simulink model "flightControlSystem"  (R2024b)
settings: Solver=ode3  StartTime=0  StopTime=TFinal  FixedStep=Ts  RelTol=1e-3  EnableMultiTasking=on
undefined symbols (not defined in the file): codertarget, Controller, DiscIntNeverNeededParam, Discrete, Estimator, g, gray, init, orient_ref, pos_ref, Sensors, Time, Ts, var_acc_angle_N, var_bias_gyr_N, var_gyro_p_N, Vehicle
libraries: simulink x42, slpidlib x6, simulink_extras x5, ctrlSharedLib x4, sharedtransform x3, visiontransforms x2, parrotlib x1, vrlib x1, visionanalysis x1, visionstatistics x1, visionconversions x1
(part 3 of 3)

== system flightControlSystem/Control System/State Estimator/SensorPreprocessing/sensordata_group ==
  HAL_acc_SI : Inport  OutDataTypeStr=Bus: HAL_acc_SI_t
  HAL_gyro_SI : Inport  Port=2  OutDataTypeStr=Bus: HAL_gyro_SI_t
  HAL_ultrasound_SI : Inport  Port=3  OutDataTypeStr=Bus: HAL_ultrasound_SI_t
  HAL_pressure_SI : Inport  Port=4  OutDataTypeStr=Bus: HAL_pressure_SI_t
  HAL_vbat_SI : Inport  Port=5  OutDataTypeStr=Bus: HAL_vbat_SI_t
  Bus Selector1 : BusSelector  OutputSignals=vbat_V,vbat_percentage
  Bus Selector3 : BusSelector  OutputSignals=x,y,z
  Bus Selector4 : BusSelector  OutputSignals=x,y,z,temperature
  Bus Selector5 : BusSelector  OutputSignals=altitude
  Bus Selector6 : BusSelector  OutputSignals=pressure
  Out Bus Element : Outport  VectorParamsAs1DForOutWhenUnconnected=off  PortName=sensordata_datin  Element=ddx
  Out Bus Element1 : Outport  VectorParamsAs1DForOutWhenUnconnected=off  PortName=sensordata_datin  Element=ddy
  Out Bus Element2 : Outport  VectorParamsAs1DForOutWhenUnconnected=off  PortName=sensordata_datin  Element=ddz
  Out Bus Element3 : Outport  VectorParamsAs1DForOutWhenUnconnected=off  PortName=sensordata_datin  Element=p
  Out Bus Element4 : Outport  VectorParamsAs1DForOutWhenUnconnected=off  PortName=sensordata_datin  Element=q
  Out Bus Element5 : Outport  VectorParamsAs1DForOutWhenUnconnected=off  PortName=sensordata_datin  Element=r
  Out Bus Element6 : Outport  VectorParamsAs1DForOutWhenUnconnected=off  PortName=sensordata_datin  Element=altitude_sonar
  Out Bus Element7 : Outport  VectorParamsAs1DForOutWhenUnconnected=off  PortName=sensordata_datin  Element=prs
  Out Bus Element8 : Outport  VectorParamsAs1DForOutWhenUnconnected=off  PortName=sensordata_datin  Element=vbat_V
  Out Bus Element9 : Outport  VectorParamsAs1DForOutWhenUnconnected=off  PortName=sensordata_datin  Element=vbat_percentage
  Out1 : Outport  Port=2
  wires:
  HAL_gyro_SI/1 -> Bus Selector4/1
  HAL_acc_SI/1 -> Bus Selector3/1
  HAL_pressure_SI/1 -> Bus Selector6/1
  HAL_ultrasound_SI/1 -> Bus Selector5/1
  Bus Selector4/1 -> Out Bus Element3/1  "<x>"
  Bus Selector3/3 -> Out Bus Element2/1  "<z>"
  Bus Selector4/3 -> Out Bus Element5/1  "<z>"
  Bus Selector5/1 -> Out Bus Element6/1  "<altitude>"
  Bus Selector6/1 -> Out Bus Element7/1  "<pressure>"
  Bus Selector4/2 -> Out Bus Element4/1  "<y>"
  Bus Selector3/1 -> Out Bus Element/1  "<x>"
  Bus Selector3/2 -> Out Bus Element1/1  "<y>"
  Bus Selector1/1 -> Out Bus Element8/1  "<vbat_V>"
  HAL_vbat_SI/1 -> Bus Selector1/1
  Bus Selector1/2 -> Out Bus Element9/1  "<vbat_percentage>"
  Bus Selector4/4 -> Out1/1  "<temperature>"

== system flightControlSystem/Control System/State Estimator/XY Position Estimator/EstimatorVelocity ==
  opticalFlow_datin : Inport
  Z_estimin : Inport  Port=2  SampleTime=Ts
  sensorIMU_datin : Inport  Port=3
  orient_estimin : Inport  Port=4
  angular velocity : Inport  Port=5
  AccelerationHandling : Subsystem
  Angular velocity compensation for optical flow : Subsystem
  DataHandling : Subsystem
  Delay : Delay  DelayLength=1  InitialCondition=0
  KalmanFilter_dxdy : ctrlSharedLib/Kalman Filter  TimeDomain=Discrete-Time  UseCurrentEstimator=on  ModelSource=Individual A, B, C, D matrices  ModelSourceVariable=ss(0.95,1,1,0,1)  A=Estimator.pos.kfVelo.A  B=Estimator.pos.kfVelo.B  C=Estimator.pos.kfVelo.C  D=Estimator.pos.kfVelo.D  NumberOfStates=1  NumberOfInputs=1  NumberOfOutputs=1  InitialEstimateSource=Dialog  X0=0  P0=10  UseK=off  UseGH=off  NumberOfProcessNoiseInputs=1  G=Estimator.pos.kfVelo.G  TimeInvariantG=on  H=Estimator.pos.kfVelo.H  TimeInvariantH=on  Q=Estimator.pos.kfVelo.Q  TimeInvariantQ=on  R=Estimator.pos.kfVelo.R  TimeInvariantR=on  N=Estimator.pos.kfVelo.N  TimeInvariantN=on  AddInputPort=on  AddEnablePort=on  OutputEstimatedY=off  OutputP=off  Ts=-1
  Selector1 : Selector  InputPortWidth=4  IndexOptions=Index vector (dialog)  Indices=[1 2]  OutputSizes=1
  Z_estimin1 : InportShadow  Port=2  SampleTime=Ts
  angular velocity compensation : Sum
  xy velocity w/o angular velocity compensation : Subsystem
  dxy_estimout : Outport  VectorParamsAs1DForOutWhenUnconnected=off
  wires:
  Z_estimin/1 -> DataHandling/1(Z_estimin), AccelerationHandling/4(Z_estimin)
  KalmanFilter_dxdy/1 -> Selector1/1
  sensorIMU_datin/1 -> AccelerationHandling/2(sensorIMU_datin), DataHandling/3(sensorIMU_datin)
  orient_estimin/1 -> AccelerationHandling/3(orient_estimin), DataHandling/2(orient_estimin)
  Z_estimin1/1 -> xy velocity w/o angular velocity compensation/2(z_estimate), Angular velocity compensation for optical flow/1(z_estimate)
  AccelerationHandling/1(acceleration_world) -> KalmanFilter_dxdy/1
  angular velocity compensation/1 -> KalmanFilter_dxdy/2
  Delay/1 -> DataHandling/5(dxyOF_datin)
  Selector1/1 -> dxy_estimout/1, Delay/1
  angular velocity/1 -> Angular velocity compensation for optical flow/2(Angular velocity w/o bias)
  Angular velocity compensation for optical flow/1(angular velocity correction) -> angular velocity compensation/2
  xy velocity w/o angular velocity compensation/1(optical_flow_dx_dy) -> DataHandling/4(dxy_estimin), AccelerationHandling/1(dxy_estimin), angular velocity compensation/1
  opticalFlow_datin/1 -> xy velocity w/o angular velocity compensation/1(optical_flow)
  DataHandling/1(enable_flag) -> KalmanFilter_dxdy/3

== system flightControlSystem/Control System/State Estimator/XY Position Estimator/EstimatorXYPosition ==
  note: Switching from orientationControl to Position
      | control reset the current world position estimate
      | (happens when using no markers)
  dxy_estimin : Inport
  orient_estimin : Inport  Port=2  SampleTime=Ts
  controlModePosVSOrient_flagin : Inport  Port=3
  dz_estimin : Inport  Port=4
  Math Function : Math  Operator=transpose  SignedPower=on
  Mux2 : Mux  Inputs=2
  Product : Product  Multiplication=Matrix(*)
  Rotation Angles to Direction Cosine Matrix : sharedtransform/Rotation Angles to Direction Cosine Matrix  rotationOrder=ZYX  aMode=aMode
  SelectdXY : Selector  InputPortWidth=3  IndexOptions=Index vector (dialog)  Indices=[1 2]  OutputSizes=1
  SimplyIntegrateVelocity : DiscreteIntegrator  ExternalReset=rising  SampleTime=Ts  ICPrevOutput=DiscIntNeverNeededParam  ICPrevScaledInput=DiscIntNeverNeededParam
  XY_estimout : Outport  VectorParamsAs1DForOutWhenUnconnected=off
  wires:
  controlModePosVSOrient_flagin/1 -> SimplyIntegrateVelocity/2
  Product/1 -> SelectdXY/1
  Mux2/1 -> Product/2
  dz_estimin/1 -> Mux2/2
  SimplyIntegrateVelocity/1 -> XY_estimout/1
  dxy_estimin/1 -> Mux2/1
  orient_estimin/1 -> Rotation Angles to Direction Cosine Matrix/1
  Rotation Angles to Direction Cosine Matrix/1 -> Math Function/1
  SelectdXY/1 -> SimplyIntegrateVelocity/1
  Math Function/1 -> Product/1

== system flightControlSystem/Control System/State Estimator/SensorPreprocessing/Temperature Compensation/Triggered Subsystem ==
  In1 : Inport
  Trigger : TriggerPort  TriggerType=either  VariantControl=Variant
  Out1 : Outport
  wires:
  In1/1 -> Out1/1

== system flightControlSystem/Control System/State Estimator/XY Position Estimator/EstimatorVelocity/AccelerationHandling ==
  dxy_estimin : Inport
  sensorIMU_datin : Inport  Port=2
  orient_estimin : Inport  Port=3
  Z_estimin : Inport  Port=4
  Add : Sum  Inputs=-+
  Bus Selector1 : BusSelector  OutputSignals=ddx,ddy,ddz
  Deactivate Acceleration If OF is not used due to low altitude : simulink/Logic and Bit Operations/Compare To Constant  relop=<=  const=Estimator.pos.opticalFlowZMax  OutDataTypeStr=boolean
  Logical Operator : Logic  Operator=OR  AllPortsSameDT=off  OutDataTypeStr=boolean
  Mux6 : Mux  Inputs=3
  Product : Product  Inputs=3
  Product1 : Product  Multiplication=Matrix(*)
  Rotation Angles to Direction Cosine Matrix : sharedtransform/Rotation Angles to Direction Cosine Matrix  rotationOrder=ZYX  aMode=aMode
  SelectPlanarddxy : Selector  InputPortWidth=3  IndexOptions=Index vector (dialog)  Indices=[1 2]  OutputSizes=1
  Selector : Selector  InputPortWidth=2  IndexOptions=Index vector (dialog)  Indices=1  OutputSizes=1
  Selector1 : Selector  InputPortWidth=2  IndexOptions=Index vector (dialog)  Indices=2  OutputSizes=1
  do not use acc if optical flow never available (Note OF@60Hz but ZOH to 200!) : simulink/Logic and Bit Operations/Compare To Constant  relop=~=  const=0  OutDataTypeStr=boolean
  do not use acc if optical flow never available (Note OF@60Hz but ZOH to 200!)1 : simulink/Logic and Bit Operations/Compare To Constant  relop=~=  const=0  OutDataTypeStr=boolean
  gainaccinput1 : Gain  OutDataTypeStr=single
  gravity : Constant  Value=[0 0 -g]
  acceleration_world : Outport  OutDataTypeStr=single  VectorParamsAs1DForOutWhenUnconnected=off
  wires:
  do not use acc if optical flow never available (Note OF@60Hz but ZOH to 200!)1/1 -> Logical Operator/2
  do not use acc if optical flow never available (Note OF@60Hz but ZOH to 200!)/1 -> Logical Operator/1
  Logical Operator/1 -> Product/1
  Selector1/1 -> do not use acc if optical flow never available (Note OF@60Hz but ZOH to 200!)1/1
  Selector/1 -> do not use acc if optical flow never available (Note OF@60Hz but ZOH to 200!)/1
  dxy_estimin/1 -> Selector1/1, Selector/1
  Product/1 -> acceleration_world/1
  Deactivate Acceleration If OF is not used due to low altitude/1 -> Product/3
  Z_estimin/1 -> Deactivate Acceleration If OF is not used due to low altitude/1
  Add/1 -> SelectPlanarddxy/1
  Product1/1 -> Add/1
  gravity/1 -> Product1/2
  SelectPlanarddxy/1 -> gainaccinput1/1
  Bus Selector1/3 -> Mux6/3  "<ddz>"
  Bus Selector1/1 -> Mux6/1  "<ddx>"
  sensorIMU_datin/1 -> Bus Selector1/1
  Mux6/1 -> Add/2
  Bus Selector1/2 -> Mux6/2  "<ddy>"
  orient_estimin/1 -> Rotation Angles to Direction Cosine Matrix/1
  Rotation Angles to Direction Cosine Matrix/1 -> Product1/1
  gainaccinput1/1 -> Product/2

== system flightControlSystem/Control System/State Estimator/XY Position Estimator/EstimatorVelocity/Angular velocity compensation for optical flow ==
  note: Optical flow readings are affected by both linear and angular velocity of the drone. We need to subtract the effect of angular velocity before using the flow data
  z_estimate : Inport
  Angular velocity w/o bias : Inport  Port=2
  Abs : Abs  SaturateOnIntegerOverflow=off
  Data Type Conversion : DataTypeConversion  SaturateOnIntegerOverflow=off  RndMeth=Floor
  Demux : Demux  Outputs=2
  Gain1 : Gain  Gain=-1
  Mux : Mux  Inputs=2
  Selector : Selector  InputPortWidth=3  IndexOptions=Index vector (dialog)  Indices=[1 2]  OutputSizes=1
  prod : Product  Inputs=**
  angular velocity correction : Outport
  wires:
  Gain1/1 -> Mux/1
  Mux/1 -> Data Type Conversion/1
  Demux/2 -> Gain1/1
  Data Type Conversion/1 -> angular velocity correction/1
  prod/1 -> Demux/1
  z_estimate/1 -> Abs/1
  Demux/1 -> Mux/2
  Selector/1 -> prod/2
  Abs/1 -> prod/1
  Angular velocity w/o bias/1 -> Selector/1

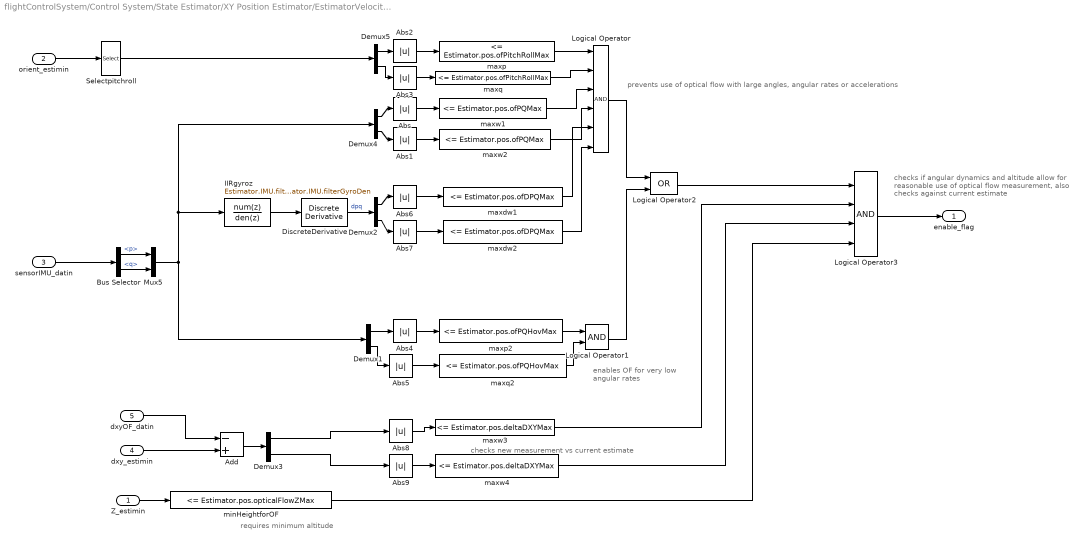
== system flightControlSystem/Control System/State Estimator/XY Position Estimator/EstimatorVelocity/DataHandling ==
  note: prevents use of optical flow with large angles, angular rates or accelerations
  note: enables OF for very
      | low angular rates
  note: checks if angular dynamics and altitude allow for
      | reasonable use of optical flow measurement,
      | also checks against current estimate
  note: checks new measurement vs current estimate
  note: requires minimum altitude
  Z_estimin : Inport
  orient_estimin : Inport  Port=2
  sensorIMU_datin : Inport  Port=3
  dxy_estimin : Inport  Port=4
  dxyOF_datin : Inport  Port=5
  Abs{,1..9} (10 alike) : Abs  SaturateOnIntegerOverflow=off
  Add : Sum  Inputs=-+
  Bus Selector : BusSelector  OutputSignals=p,q
  Demux{1..5} (5 alike) : Demux  Outputs=2
  DiscreteDerivative : simulink/Discrete/Discrete Derivative  gainval=1.0  ICPrevScaledInput=0.0  OutMin=[]  OutMax=[]  OutDataType=fixdt(1, 16)  OutScaling=2^-10  DoSatur=off
  IIRgyroz : DiscreteFilter  Numerator=Estimator.IMU.filterGyroNum  Denominator=Estimator.IMU.filterGyroDen
  Logical Operator : Logic  Inputs=6  AllPortsSameDT=off  OutDataTypeStr=boolean
  Logical Operator1 : Logic  AllPortsSameDT=off  OutDataTypeStr=boolean
  Logical Operator2 : Logic  Operator=OR  AllPortsSameDT=off  OutDataTypeStr=boolean
  Logical Operator3 : Logic  Inputs=4  AllPortsSameDT=off  OutDataTypeStr=boolean
  Mux5 : Mux  Inputs=2
  Selectpitchroll : Selector  InputPortWidth=3  IndexOptions=Index vector (dialog)  Indices=[2 3]  OutputSizes=1
  maxdw1 : simulink/Logic and Bit Operations/Compare To Constant  relop=<=  const=Estimator.pos.ofDPQMax  OutDataTypeStr=boolean
  maxdw2 : simulink/Logic and Bit Operations/Compare To Constant  relop=<=  const=Estimator.pos.ofDPQMax  OutDataTypeStr=boolean
  maxp : simulink/Logic and Bit Operations/Compare To Constant  relop=<=  const=Estimator.pos.ofPitchRollMax  OutDataTypeStr=boolean
  maxp2 : simulink/Logic and Bit Operations/Compare To Constant  relop=<=  const=Estimator.pos.ofPQHovMax  OutDataTypeStr=boolean
  maxq : simulink/Logic and Bit Operations/Compare To Constant  relop=<=  const=Estimator.pos.ofPitchRollMax  OutDataTypeStr=boolean
  maxq2 : simulink/Logic and Bit Operations/Compare To Constant  relop=<=  const=Estimator.pos.ofPQHovMax  OutDataTypeStr=boolean
  maxw1 : simulink/Logic and Bit Operations/Compare To Constant  relop=<=  const=Estimator.pos.ofPQMax  OutDataTypeStr=boolean
  maxw2 : simulink/Logic and Bit Operations/Compare To Constant  relop=<=  const=Estimator.pos.ofPQMax  OutDataTypeStr=boolean
  maxw3 : simulink/Logic and Bit Operations/Compare To Constant  relop=<=  const=Estimator.pos.deltaDXYMax  OutDataTypeStr=boolean
  maxw4 : simulink/Logic and Bit Operations/Compare To Constant  relop=<=  const=Estimator.pos.deltaDXYMax  OutDataTypeStr=boolean
  minHeightforOF : simulink/Logic and Bit Operations/Compare To Constant  relop=<=  const=Estimator.pos.opticalFlowZMax  OutDataTypeStr=boolean
  enable_flag : Outport  VectorParamsAs1DForOutWhenUnconnected=off
  wires:
  minHeightforOF/1 -> Logical Operator3/4
  IIRgyroz/1 -> DiscreteDerivative/1
  Mux5/1 -> Demux1/1, Demux4/1, IIRgyroz/1
  maxw4/1 -> Logical Operator3/3
  maxw3/1 -> Logical Operator3/2
  dxyOF_datin/1 -> Add/1
  Demux3/2 -> Abs9/1
  Demux3/1 -> Abs8/1
  dxy_estimin/1 -> Add/2
  Add/1 -> Demux3/1
  Abs9/1 -> maxw4/1
  Abs8/1 -> maxw3/1
  Logical Operator2/1 -> Logical Operator3/1
  Logical Operator3/1 -> enable_flag/1
  DiscreteDerivative/1 -> Demux2/1  "dpq"
  Demux2/2 -> Abs7/1
  Demux2/1 -> Abs6/1
  Abs7/1 -> maxdw2/1
  Abs6/1 -> maxdw1/1
  Logical Operator1/1 -> Logical Operator2/2
  Demux1/2 -> Abs5/1
  Demux1/1 -> Abs4/1
  Abs5/1 -> maxq2/1
  Abs4/1 -> maxp2/1
  Abs3/1 -> maxq/1
  Abs2/1 -> maxp/1
  Demux4/2 -> Abs1/1
  Demux4/1 -> Abs/1
  Abs1/1 -> maxw2/1
  Abs/1 -> maxw1/1
  Z_estimin/1 -> minHeightforOF/1
  Logical Operator/1 -> Logical Operator2/1
  maxw1/1 -> Logical Operator/3
  Bus Selector/1 -> Mux5/1  "<p>"
  Selectpitchroll/1 -> Demux5/1
  sensorIMU_datin/1 -> Bus Selector/1
  maxq2/1 -> Logical Operator1/2
  Bus Selector/2 -> Mux5/2  "<q>"
  maxp/1 -> Logical Operator/1
  maxw2/1 -> Logical Operator/4
  orient_estimin/1 -> Selectpitchroll/1
  maxdw1/1 -> Logical Operator/5
  maxdw2/1 -> Logical Operator/6
  maxq/1 -> Logical Operator/2
  Demux5/1 -> Abs2/1
  Demux5/2 -> Abs3/1
  maxp2/1 -> Logical Operator1/1

== system flightControlSystem/Control System/State Estimator/XY Position Estimator/EstimatorVelocity/xy velocity w//o angular velocity compensation ==
  note: Optical flow raw readings are converted to velocity in m/s based on the estimated altitude
  optical_flow : Inport
  z_estimate : Inport  Port=2
  " " : Product  Inputs=**
  Compare To Constant : simulink/Logic and Bit Operations/Compare To Constant  relop=<  const=200*4  OutDataTypeStr=boolean
  Counter Free-Running : simulink/Sources/Counter Free-Running  NumBits=32  tsamp=-1
  Gain : Gain  Gain=-1
  Select dxy : Selector  InputPortWidth=3  IndexOptions=Index vector (dialog)  Indices=[1 2]  OutputSizes=1
  Switch : Switch  Criteria=u2 > Threshold  SaturateOnIntegerOverflow=off  InputSameDT=off
  opticalFlowErrorCorrect : Gain  Gain=1.15
  optical_flow_dx_dy : Outport
  wires:
  Select dxy/1 -> optical_flow_dx_dy/1  "optical_flow_dx_dy"
  " "/1 -> opticalFlowErrorCorrect/1
  opticalFlowErrorCorrect/1 -> Switch/3
  Gain/1 -> " "/2
  Switch/1 -> Select dxy/1
  Counter Free-Running/1 -> Compare To Constant/1
  Compare To Constant/1 -> Switch/2
  optical_flow/1 -> " "/1, Switch/1
  z_estimate/1 -> Gain/1

== matlab function flightControlSystem/Image Processing System/Subsystem/MATLAB Function2 ==
  data: u input; y output
function y = fcn(u)
center_row = size(u, 1) / 2; % 160 / 2 = 80
center_col = size(u, 2) / 2; % 180 / 2 = 90

% 20x20 boyutunda kesilecek alanın başlangıç koordinatları
start_row = center_row - 10; % 80 - 10 = 70
start_col = center_col - 10; % 90 - 10 = 80

% 4. 20x20 boyutunda kesilecek alanı belirleyin
cropped = imcrop(u,[0, 0, center_col, center_row]);
y = cropped;

== stateflow chart flightControlSystem/Control System/Path Planning/Chart ==
  state TakeOff
    refZ = -0.8;
    unit_vector = [0.0;0.0];
  state delay_side
  state Init
    % Birim vektör hesaplama
    refZ = -1;
    u_x = double(cos(deg2rad(yaw_degree)));
    u_y = double(sin(deg2rad(yaw_degree)));
    % Birim vektörü oluşturma
    if abs(Z) > 0.7
    unit_vector = [u_x; u_y]*0.6;
    if ~Vision_based_Data
    unit_vector = [u_x; u_y]*0.3;
    end
    else
    unit_vector = [0.0;0.0];
    end
  state Landing1
    % Birim vektörü oluşturma
    unit_vector = [0.0;0.0];
    refZ = refZ + 0.002;
    after(0.3,sec)
  state Stop
    unit_vector = [0.0;0.0];
    refZ = 0;
  (default) -> TakeOff
  TakeOff -> delay_side
  delay_side -> Init : [after(1,sec)]
  Landing1 -> Stop : [abs(Z) == 0]
  Init -> Landing1 : [abs(Z)>0.7 && landing == true]
  data: Z input; landing input; Vision_based_Data input; unit_vector output; yaw_degree input; u_y local double; u_x local double; refZ output

== matlab function flightControlSystem/Image Processing System/Subsystem/MATLAB Function3 ==
  data: u input; y output
function y = fcn(u)
center_row = size(u, 1) / 2; % 160 / 2 = 80
center_col = size(u, 2) / 2; % 180 / 2 = 90

% 20x20 boyutunda kesilecek alanın başlangıç koordinatları
start_row = center_row - 10; % 80 - 20 = 60
start_col = center_col - 10; % 90 - 20 = 70

% 4. 20x20 boyutunda kesilecek alanı belirleyin
cropped = imcrop(u,[start_col, start_row, 20, 20]);
y = cropped;

== matlab function flightControlSystem/Image Processing System/Subsystem1/Subsystem/crop_front ==
  data: u input; y output
function y = fcn(u)
%column x row
cropped = imcrop(u,[55, 1, 49, 0]);
y = cropped;

== matlab function flightControlSystem/Image Processing System/Subsystem1/Subsystem/y ==
  data: u input; y output
function y = fcn(u)
% 1 olan index'leri bul
indices = find(u == 1);

if ~isempty(indices)
    first_index = indices(1)+55;
    last_index = indices(end)+55;
    row = 1;
    intensity = size(indices);
else
    first_index = 80;
    last_index = 80;
    row = 60;
    % ağırlıklandır
    intensity = [0 0];
end
column = (first_index+last_index)/2;
y = [column, row, intensity(2)];

== matlab function flightControlSystem/Image Processing System/Subsystem1/Subsystem/crop_left ==
  data: u input; y output
function y = fcn(u)
%column x row
cropped = imcrop(u,[55, 1, 0, 49]);
y = cropped;

== matlab function flightControlSystem/Image Processing System/Subsystem1/Subsystem/crop_right ==
  data: u input; y output
function y = fcn(u)
%
cropped = imcrop(u,[105, 1, 0, 49]);
y = cropped;

== matlab function flightControlSystem/Image Processing System/Subsystem1/Subsystem/y1 ==
  data: u input; y output
function y = fcn(u)
% 1 olan index'leri bul
indices = find(u == 1);

if ~isempty(indices)
    first_index = indices(1)+0;
    last_index = indices(end)+0;
    column = 55;
    intensity = size(indices);
else
    first_index = 60;
    last_index = 60;
    column = 80;
    % ağırlıklandır
    intensity = [0 0];
end
row = (first_index+last_index)/2;
y = [column, row, intensity(1)];

== matlab function flightControlSystem/Image Processing System/Subsystem1/Subsystem/y2 ==
  data: u input; y output
function y = fcn(u)
% 1 olan index'leri bul
indices = find(u == 1);

if ~isempty(indices)
    first_index = indices(1)+0;
    last_index = indices(end)+0;
    column = 105;
    intensity = size(indices);
else
    first_index = 60;
    last_index = 60;
    column = 80;
    % ağırlıklandır
    intensity = [0 0];
end
row = (first_index+last_index)/2;
y = [column, row, intensity(1)];

== matlab function flightControlSystem/Image Processing System/Subsystem1/Subsystem/MATLAB Function ==
  data: A input; A_active output; B input; B_active output
function [A_active, B_active] = switchSignal(A, B)
% Bu fonksiyonda A ve B sinyallerine göre hangisinin aktif olacağını belirleriz.
% Başlangıçta hiçbiri aktif değilse durum=0 varsayılacaktır.
%
% İşleyiş:
% - Eğer her iki sinyal 0 ise, her ikisi pasiftir.
% - Eğer sadece bir signal 0’dan farklı ise o aktif olur.
% - Eğer her iki sinyal de 0’dan farklıysa, önceden aktif olan sinyal aktif kalır.
% - Aktif sinyal 0’ya düştüğünde, diğer sinyal 0’dan farklı ise diğer sinyal aktif olur.
%
% persistent değişken, önceki durum bilgisini saklamak için kullanılır.

persistent activeSignal; % 0: hiçbiri, 1: A aktif, 2: B aktif

if isempty(activeSignal)
    activeSignal = 0;
end

% Kendi sinyal değerlerine bakarak 0 kontrolü yapılır.
A_nonzero = (A ~= 0);
B_nonzero = (B ~= 0);

% Her iki sinyal 0 ise:
if ~A_nonzero && ~B_nonzero
    activeSignal = 0;

% Sadece A 0'dan farklı:
elseif A_nonzero && ~B_nonzero
    activeSignal = 1;

% Sadece B 0'dan farklı:
elseif ~A_nonzero && B_nonzero
    activeSignal = 2;

% Her iki sinyal 0’dan farklı durum:
else
    if activeSignal == 0
        % İlk gelen sinyal aktif olsun. Örneğin, A’ya öncelik verebilirsiniz:
        activeSignal = 1;
    else
        % Eğer aktif olan sinyal artık 0 ise, diğerini aktif yap:
        if activeSignal == 1 && ~A_nonzero
            activeSignal = 2;
        elseif activeSignal == 2 && ~B_nonzero
            activeSignal = 1;
        end
    end
end

% Aktiflik durumlarını döndür
A_active = (activeSignal == 1);
B_active = (activeSignal == 2);

== matlab function flightControlSystem/Image Processing System/MATLAB Function1 ==
  data: l input; r input; left output; right output
function [left, right]  = fcn(l, r)
if l < r
    right = 1;
    left = 0;
else
    left = 1;
    right = 0;
end

== matlab function flightControlSystem/Image Processing System/MATLAB Function2 ==
  data: R input; BW output; G input; B input
function BW = createMask(R, G, B)
% createMask  Saf kırmızı (#FF0000) rengi filtrelemek için optimize edilmiştir.
% Bu fonksiyon, kırmızı kanalının maksimumda, diğer kanalların minimumda
% olduğu pikselleri yakalar.

% 1. Kanal (Kırmızı - Red): Çok yüksek değerler (200 - 255)
channel1Min = 200.000;
channel1Max = 255.000;

% 2. Kanal (Yeşil - Green): Çok düşük değerler (0 - 40)
% Saf kırmızıda yeşil kanal 0 olmalıdır.
channel2Min = 0.000;
channel2Max = 40.000;

% 3. Kanal (Mavi - Blue): Çok düşük değerler (0 - 40)
% Saf kırmızıda mavi kanal 0 olmalıdır.
channel3Min = 0.000;
channel3Max = 40.000;

% Saf kırmızı maskesini oluştur
% Ekstra güvenlik: R kanalının hem G hem de B'den çok daha büyük olması şartını ekleyebiliriz.
sliderBW = (R >= channel1Min) & (R <= channel1Max) & ...
           (G >= channel2Min) & (G <= channel2Max) & ...
           (B >= channel3Min) & (B <= channel3Max);

BW = sliderBW;
end

== matlab function flightControlSystem/Image Processing System/Subsystem3/MATLAB Function3 ==
  data: img input; angle output
function angle = fcn(img)
redMask = img(:,:,1) > 130 & img(:,:,2) < 110 & img(:,:,3) < 110;

% 2. İSKELETLEŞTİRME (Kritik Adım)
% Kalın çizgiyi merkez hattına indirger
skel = edge(img); 

% 3. Hough Transform (İskelet üzerinden)
[H, T, R] = hough(skel);
% 'NHoodSize' parametresi ile birbirine çok yakın doğruların seçilmesini engelliyoruz
peaks = houghpeaks(H, 2, 'NHoodSize', [15 15]); 
lines = houghlines(skel, T, R, peaks, 'FillGap', 80, 'MinLength', 30);

if length(lines) >= 2
    angles = [lines(1).theta, lines(2).theta];
    angleDiff = abs(angles(1) - angles(2));
    
    % V açısı için 180 dereceye tamamlama kontrolü
    if angleDiff > 90, angleDiff = 180 - angleDiff; end

end
angle = angleDiff;

== matlab function flightControlSystem/Image Processing System/Subsystem3/MATLAB Function4 ==
  data: peaks input; angleDeg output
function angleDeg = fcn(peaks)
    % peaks: Find Local Maxima bloğundan gelen [2x2] matris
    % Örnek: [77 278; 93 267]
    if peaks ~= 0
        % 1. Parametre Tanımlama (Hough Bloğundaki değerlerle aynı olmalı)
        % Eğer blokta theta resolution pi/180 ise dTheta = 1 derecedir.
        dTheta = 1; 
        
        % 2. İndisleri Ayır (Sadece 2. sütun yani Theta indisleri lazım)
        thetaIdx1 = peaks(1, 2);
        thetaIdx2 = peaks(2, 2);
        
        % 3. İndisleri Dereceye Çevir
        % Not: Hough matrisi genellikle 1'den başlar, -90 ile 89 arası yayılır.
        theta1 = (thetaIdx1 - 1) * dTheta - 90;
        theta2 = (thetaIdx2 - 1) * dTheta - 90;
        
        % 4. Aradaki Farkı Hesapla
        angleDiff = abs(theta1 - theta2);
        
        % 5. V Şekli İçin Dar Açıyı Garantile
        if angleDiff > 90
            angleDeg = 180 - angleDiff;
        else
            angleDeg = angleDiff;
        end
    else
        angleDeg = 0;
    end
end

== matlab function flightControlSystem/Image Processing System/Subsystem3/MATLAB Function ==
  data: mask input; angle output
function angle = lineAngle(mask)
%#codegen

[rows, cols] = size(mask);
pts = zeros(rows*cols,2);
n = 0;

for i=1:rows
    for j=1:cols
        if mask(i,j)
            n = n+1;
            pts(n,:) = [j i];
        end
    end
end

if n < 10
    angle = 0;
    return;
end

pts = pts(1:n,:);

mx = mean(pts(:,1));
my = mean(pts(:,2));

x = pts(:,1) - mx;
y = pts(:,2) - my;

Sxx = sum(x.*x);
Syy = sum(y.*y);
Sxy = sum(x.*y);

theta = 0.5 * atan2(2*Sxy, Sxx - Syy);
angle = abs(theta * 180/pi);

if angle > 90
    angle = 180 - angle;
end

== matlab function flightControlSystem/Image Processing System/MATLAB Function ==
  data: u input; y output
function y = fcn(u)
center_row = size(u, 1) / 2; % 160 / 2 = 80
center_col = size(u, 2) / 2; % 180 / 2 = 90

% 20x20 boyutunda kesilecek alanın başlangıç koordinatları
start_row = center_row - 10; % 80 - 10 = 70
start_col = center_col - 10; % 90 - 10 = 80

% 4. 20x20 boyutunda kesilecek alanı belirleyin
cropped = imcrop(u,[start_col, 0, 20, 20]);
y = cropped;

== matlab function flightControlSystem/Control System/Controller/Position Controller/Position error transformation (Earth to Body frame) ==
  data: yaw input; xy_err_earth input; xy_err_body output
function xy_err_body = fcn(yaw,xy_err_earth)

transformation = [cos(yaw), sin(yaw); -sin(yaw),  cos(yaw)];
xy_err_body = transformation * xy_err_earth;


end

== matlab function flightControlSystem/Control System/Path Planning/modulo ==
  data: u input; y output
function y = fcn(u)
if u < 0
    y = (mod(u, 360) - 360); % Negatif değerler için düzeltme cw
else
    y = mod(u, 360); % 0-360 aralığına sarmak için mod işlemi ccw
end

%%
% function y = map_angle(n)
%     y = mod(n, 360); % 0-360 aralığına sarmak için mod işlemi
%     if y < 0
%         y = y + 360; % Negatif değerler için düzeltme
%     end
% end
%%

== matlab function flightControlSystem/Image Processing System/Subsystem/MATLAB Function1 ==
  data: u input; y output
function y = fcn(u)
center_row = size(u, 1) / 2; % 160 / 2 = 80
center_col = size(u, 2) / 2; % 180 / 2 = 90

% 20x20 boyutunda kesilecek alanın başlangıç koordinatları
start_row = center_row - 10; % 80 - 10 = 70
start_col = center_col - 10; % 90 - 10 = 80

% 4. 20x20 boyutunda kesilecek alanı belirleyin
cropped = imcrop(u,[center_col, 0, size(u, 2), center_row]);
y = cropped;
